simulink model "REALY_UNIT_TEST"  (Simulink 7.8)
settings: Solver=ode4  StartTime=0.0  StopTime=1.2  FixedStep=Ts  MaxStep=1e-3  RelTol=1e-3
model workspace (MAT data in the model file):
  op_snapshot1 : opcond.OperatingPoint (value not decoded)
PostLoadFcn:
  | Ts=80e-6;
InitFcn:
  | Ts=80e-6;
libraries: powerlib x5, modbus_lib x4, cables_lib x3, artemis x1, dynamic_load_lib x1, simulink x1
settings Model: ARTEMISmethode_block_infos=$$__separator__$$REALY_UNIT_TEST/ARTEMIS Guide$$__separator__$$  Creator=RE25624  LastModifiedBy=re25624  BufferReuse=off
settings SolverCC: ZeroCrossAlgorithm=Adaptive
settings DataIOCC: ExternalInput=getinputstruct(op_snapshot1)  InitialState=getstatestruct(op_snapshot1)  LimitDataPoints=off  MaxDataPoints=90060  SignalLoggingSaveFormat=Dataset  SaveOutput=off  SignalLogging=off  DSMLogging=off  SaveTime=off  OutputSaveName=result
settings OptimizationCC: BlockReduction=off  OptimizeBlockIOStorage=off  BufferReuse=off  ExpressionFolding=off  LocalBlockOutputs=off
settings DebuggingCC: MaxConsecutiveZCsMsg=warning  IgnoredZcDiagnostic=none  SolverPrmCheckMsg=none  MultiTaskRateTransMsg=warning  FrameProcessingCompatibilityMsg=error  ModelReferenceExtraNoncontSigs=warning  StrictBusMsg=None
settings ModelReferenceCC: UpdateModelReferenceTargets=IfOutOfDate
settings SFSimCC: SFSimEcho=off
settings GRTTargetCC: TargetFunctionLibrary=C89/C90 (ANSI)

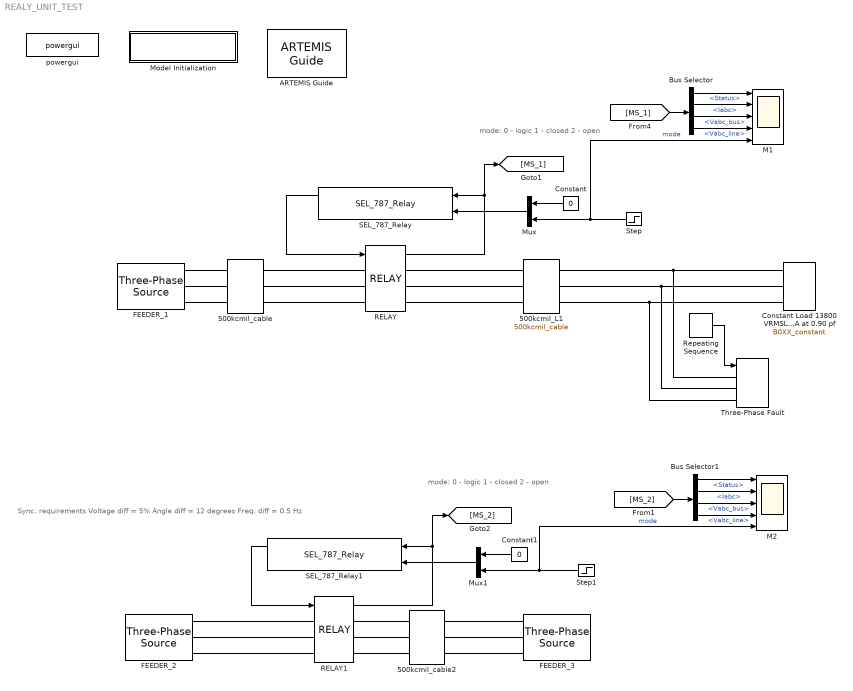
== system REALY_UNIT_TEST ==
  note: mode:
      | 0 - logic
      | 1 - closed
      | 2 - open
  note: mode:
      | 0 - logic
      | 1 - closed
      | 2 - open
  note: Sync. requirements
      | Voltage diff = 5%
      | Angle diff = 12 degrees
      | Freq. diff = 0.5 Hz
  500kcmil_L1 : cables_lib/500kcmil_cable  length=2000  par_sets=1
  500kcmil_cable : cables_lib/500kcmil_cable  length=13000  par_sets=1
  500kcmil_cable2 : cables_lib/500kcmil_cable  length=30000  par_sets=1
  ARTEMIS Guide : artemis/ARTEMIS/ARTEMIS Guide  Tag=FTSSmethode_opal_4hx0r99  Description=5.0_z1  lock=on  Ts=Ts  opt=art5  dyna=off  nb_perm=4  RT_fullcomp=off  ssn=on  ssn_itvc=off  ssn_ivic=off  ssn_ext=off  ssn_solver=Art5 with Backward Euler nodal interface  ssn_impulse=off  ssn_quasimpulse=off  ssn_impulse_loop=2  paraExtinctionThy=off  Thy_Impulse=on  dtc=Off  dtc_opt=normal  ao=on  simtype=off  ct_mac=off  lin_mov=off  lsp=[0.001 2]  spike_skip=Disabled  dtc_extra=1  dtc_sws=normal  dtc_pied=0.5  SPSRulesBlock=SPSRules  tre=on  ctmm=off  LF=off  dpl_type=ARTEMiS DPL  rlc_type=off  custom_type=off  para=on  ssn_ImpulseLoopBlockedStateUpdate=2  ssn_mov_iter_number=5  ssn_switch_iter_number=5
  Bus Selector : BusSelector  OutputSignals=Status,Iabc,Vabc_bus,Vabc_line
  Bus Selector1 : BusSelector  OutputSignals=Status,Iabc,Vabc_bus,Vabc_line
  Constant : Constant  Value=0
  Constant Load 13800 VRMSLL 5000 kVA at 0.90 pf : dynamic_load_lib/B0XX_constant  v=13800  kVA=10000  pf=0.85
  Constant1 : Constant  Value=0
  FEEDER_1 : powerlib/Electrical Sources/Three-Phase Source  Voltage=13800  PhaseAngle=0  Frequency=60  InternalConnection=Yg  SpecifyImpedance=on  Resistance=0.8929  Inductance=16.58e-3  ShortCircuitLevel=375e6  BaseVoltage=13800  XRratio=7.9  BusType=swing  Pref=0  Qref=0  Qmin=-inf  Qmax=inf
  FEEDER_2 : powerlib/Electrical Sources/Three-Phase Source  Voltage=13800  PhaseAngle=0  Frequency=60  InternalConnection=Yg  SpecifyImpedance=on  Resistance=0.8929  Inductance=16.58e-3  ShortCircuitLevel=375e6  BaseVoltage=13800  XRratio=7.9  BusType=swing  Pref=0  Qref=0  Qmin=-inf  Qmax=inf
  FEEDER_3 : powerlib/Electrical Sources/Three-Phase Source  Voltage=13800*1.04  PhaseAngle=-10  Frequency=60  InternalConnection=Yg  SpecifyImpedance=on  Resistance=0.8929  Inductance=16.58e-3  ShortCircuitLevel=375e6  BaseVoltage=13800  XRratio=7.9  BusType=swing  Pref=0  Qref=0  Qmin=-inf  Qmax=inf
  M1 : Scope  NumInputPorts=5
      settings: TimeRange=1.4  YMin=0~-15000~-30000~-50000~0  YMax=1~15000~50000~30000~1
  M2 : Scope  NumInputPorts=5
      settings: TimeRange=1.4  YMin=0~-4000~-15000~-15000~1  YMax=1~4000~15000~15000~2
  Model Initialization : Subsystem  AncestorBlock=artemis/Tools /Misc/Model Initialization  mask(Model Functions){InitFcnX=Ts=80e-6;, prel=off, posl=on, inif=on, strf=off}
      mask prompts: InitFcnX "Initialisation"; prel "Preload Function"; posl "PostLoad Function"; inif "InitFcn"; strf "StartFcn"
      mask init:
      | currentBlock = gcb;
      | root = bdroot(currentBlock);
      | 
      | if ~strcmp(get_param(root,'BlockDiagramType'),'library')
      |     if prel==1
      |         set_param(root, 'PreLoadFcn', InitFcnX);
      |     else
      |         set_param(root, 'PreLoadFcn', '');
      |     end
      |     if inif==1
      |         set_param(root, 'InitFcn', InitFcnX);
      |     else
      |         set_param(root, 'InitFcn', '');
      |     end
      |     if strf==1
      |         set_param(root, 'StartFcn', InitFcnX);
      |     else
      |         set_param(root, 'StartFcn', '');
      |     end
      |     if posl==1
      |         set_param(root, 'PostLoadFcn', InitFcnX);
      |     else
      |         set_param(root, 'PostLoadFcn', '');
      |     end
      | end
      | 
      | pos = get_param(currentBlock, 'Position');
      | width = pos(3) - pos(1); height = pos(4) - pos(2);
      | txt = [ upper(root) '\n' '- InitFcn. . . . . '  get_param(root, 'InitFcn') ];
      settings: CopyFcn=set_param(gcb,'LinkStatus','inactive')
      mask Display: text(5, height*0.5, txt, 'horizontalAlignment', 'left', 'verticalAlignment', 'middle') ;
  Mux : Mux  Inputs=2
  Mux1 : Mux  Inputs=2
  RELAY : modbus_lib/RELAY  Ts=Ts
      link override Three-Phase V-I Measurement/Model/VI/Ia: GotoTag=LibraryTag_Ia
      link override Three-Phase V-I Measurement/Model/VI/Ib: GotoTag=LibraryTag_Ib
      link override Three-Phase V-I Measurement/Model/VI/Ic: GotoTag=LibraryTag_Ic
      link override Three-Phase V-I Measurement/Model/VI/Va: GotoTag=LibraryTag_Va
      link override Three-Phase V-I Measurement/Model/VI/Vb: GotoTag=LibraryTag_Vb
      link override Three-Phase V-I Measurement/Model/VI/Vc: GotoTag=LibraryTag_Vc
      link override Three-Phase V-I Measurement1/Model/VI/Ia: GotoTag=LibraryTag_Ia
      link override Three-Phase V-I Measurement1/Model/VI/Ib: GotoTag=LibraryTag_Ib
      link override Three-Phase V-I Measurement1/Model/VI/Ic: GotoTag=LibraryTag_Ic
      link override Three-Phase V-I Measurement1/Model/VI/Va: GotoTag=LibraryTag_Va
      link override Three-Phase V-I Measurement1/Model/VI/Vb: GotoTag=LibraryTag_Vb
      link override Three-Phase V-I Measurement1/Model/VI/Vc: GotoTag=LibraryTag_Vc
  RELAY1 : modbus_lib/RELAY  Ts=Ts
      link override Three-Phase V-I Measurement/Model/VI/Ia: GotoTag=LibraryTag_Ia
      link override Three-Phase V-I Measurement/Model/VI/Ib: GotoTag=LibraryTag_Ib
      link override Three-Phase V-I Measurement/Model/VI/Ic: GotoTag=LibraryTag_Ic
      link override Three-Phase V-I Measurement/Model/VI/Va: GotoTag=LibraryTag_Va
      link override Three-Phase V-I Measurement/Model/VI/Vb: GotoTag=LibraryTag_Vb
      link override Three-Phase V-I Measurement/Model/VI/Vc: GotoTag=LibraryTag_Vc
      link override Three-Phase V-I Measurement1/Model/VI/Ia: GotoTag=LibraryTag_Ia
      link override Three-Phase V-I Measurement1/Model/VI/Ib: GotoTag=LibraryTag_Ib
      link override Three-Phase V-I Measurement1/Model/VI/Ic: GotoTag=LibraryTag_Ic
      link override Three-Phase V-I Measurement1/Model/VI/Va: GotoTag=LibraryTag_Va
      link override Three-Phase V-I Measurement1/Model/VI/Vb: GotoTag=LibraryTag_Vb
      link override Three-Phase V-I Measurement1/Model/VI/Vc: GotoTag=LibraryTag_Vc
  Repeating Sequence : simulink/Sources/Repeating Sequence  rep_seq_t=[0 0.05 0.05 0.9 0.9 4]  rep_seq_y=[0 0 1 1 0 0]
  SEL_787_Relay : modbus_lib/SEL_787_Relay  bkrCtrl_enable=0  bkrCtrl_status=1  settings=[13800, 40000, 150, 5, 12, 0.5]  Ts=Ts
  SEL_787_Relay1 : modbus_lib/SEL_787_Relay  bkrCtrl_enable=0  bkrCtrl_status=1  settings=[13800, 40000, 150, 5, 12, 0.5]  Ts=Ts
  Step : Step  SampleTime=Ts
  Step1 : Step  Time=0.6  Before=2  SampleTime=Ts
  Three-Phase Fault : powerlib/Elements/Three-Phase Fault  FaultA=on  FaultB=on  FaultC=on  FaultResistance=1e-4  GroundFault=on  GroundResistance=1e-4  External=on  SwitchStatus=[1 0]  SwitchTimes=[ 1/60 5/60]  InitialStates=[0 0 0]  SnubberResistance=1e6  SnubberCapacitance=inf  Measurements=None
  powergui : powerlib/powergui  Priority=2  SimulationMode=Discrete  SolverType=Tustin  SampleTime=Ts  frequency=60  SPID=off  DisableSnubberDevices=off  DisableRonSwitches=off  DisableVfSwitches=off  SwTol=0  Interpol=off  DisplayEquations=off  FunctionMessages=off  frequencyindice=0  Pbase=100e6  ErrMax=1e-4  Iterations=50  UnitsV=kV  UnitsW=MW  echomessages=off  HookPort=off  EnableUseOfTLC=off  x0status=blocks  RestoreLinks=warning  ResistiveCurrentMeasurement=off  Frange=logspace(0,3,50)  Ylog=off  Xlog=off  ShowGrid=off  save=off  variable=ZData  structure=0  ZoomFFT=on  StartTime=0.0  cycles=2  DisplayStyle=off  fundamental=60  FreqAxis=off  MaxFrequency=1000  frequencyindicesteady=1  RmsSteady=1  display=off  Ts=0  methode=off
  wires:
  [MS_1] -> Bus Selector/1
  Step/1 -> Mux/2, M1/5  "mode"
  RELAY/1 -> [MS_1], SEL_787_Relay/1
  SEL_787_Relay/1 -> RELAY/1
  Mux/1 -> SEL_787_Relay/2
  Bus Selector/1 -> M1/1  "<Status>"
  Bus Selector/2 -> M1/2  "<Iabc>"
  Bus Selector/3 -> M1/3  "<Vabc_bus>"
  Bus Selector/4 -> M1/4  "<Vabc_line>"
  Constant/1 -> Mux/1
  Repeating Sequence/1 -> Three-Phase Fault/1
  [MS_2] -> Bus Selector1/1
  Step1/1 -> Mux1/2, M2/5  "mode"
  RELAY1/1 -> [MS_2], SEL_787_Relay1/1
  SEL_787_Relay1/1 -> RELAY1/1
  Mux1/1 -> SEL_787_Relay1/2
  Bus Selector1/1 -> M2/1  "<Status>"
  Bus Selector1/2 -> M2/2  "<Iabc>"
  Bus Selector1/3 -> M2/3  "<Vabc_bus>"
  Bus Selector1/4 -> M2/4  "<Vabc_line>"
  Constant1/1 -> Mux1/1
  connections:
  500kcmil_cable/LConn1 -- FEEDER_1/RConn1
  500kcmil_cable/LConn2 -- FEEDER_1/RConn2
  500kcmil_cable/LConn3 -- FEEDER_1/RConn3
  Constant Load 13800 VRMSLL 5000 kVA at 0.90 pf/LConn3 -- Three-Phase Fault/LConn3 -- 500kcmil_L1/RConn3
  Constant Load 13800 VRMSLL 5000 kVA at 0.90 pf/LConn2 -- Three-Phase Fault/LConn2 -- 500kcmil_L1/RConn2
  Constant Load 13800 VRMSLL 5000 kVA at 0.90 pf/LConn1 -- Three-Phase Fault/LConn1 -- 500kcmil_L1/RConn1
  RELAY/RConn3 -- 500kcmil_L1/LConn3
  RELAY/RConn2 -- 500kcmil_L1/LConn2
  RELAY/RConn1 -- 500kcmil_L1/LConn1
  500kcmil_cable/RConn3 -- RELAY/LConn3
  500kcmil_cable/RConn2 -- RELAY/LConn2
  500kcmil_cable/RConn1 -- RELAY/LConn1
  RELAY1/LConn3 -- FEEDER_2/RConn3
  RELAY1/LConn2 -- FEEDER_2/RConn2
  RELAY1/LConn1 -- FEEDER_2/RConn1
  FEEDER_3/RConn3 -- 500kcmil_cable2/LConn3
  FEEDER_3/RConn2 -- 500kcmil_cable2/LConn2
  FEEDER_3/RConn1 -- 500kcmil_cable2/LConn1
  500kcmil_cable2/RConn3 -- RELAY1/RConn3
  500kcmil_cable2/RConn2 -- RELAY1/RConn2
  500kcmil_cable2/RConn1 -- RELAY1/RConn1

== system REALY_UNIT_TEST/Model Initialization ==
